simulink model "test_buoy_detector"  (Simulink 7.6)
settings: Solver=FixedStepDiscrete  StartTime=0.0  StopTime=0  RelTol=1e-3
undefined symbols (not defined in the file or in its folder): gray, jet, Rec, Scale_Forward_B, Scale_Forward_G, Scale_Forward_H, Scale_Forward_R, Scale_Forward_S, Scale_Forward_V, SDTV
libraries: vipsnks x10, vipconversions x3, viptextngfix x2, vipsrcs x1, dspmtrx3 x1
settings Model: Creator=Thing 1  LastModifiedBy=auvt
settings RTWCC: TargetLang=C++

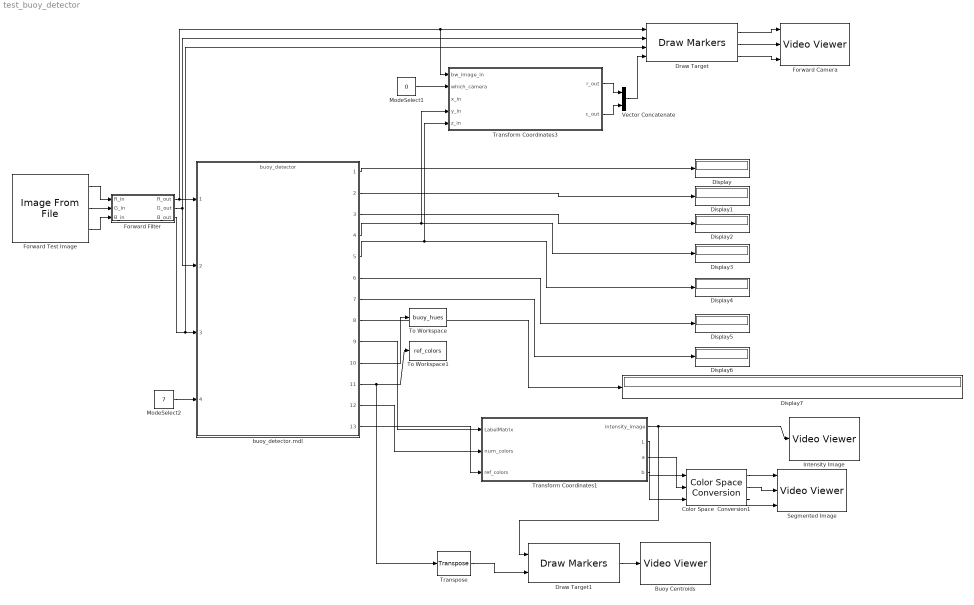
== system test_buoy_detector ==
  Buoy Centroids : vipsnks/Video Viewer  DialogControllerArgs=DataTag1  inputType=Obsolete7b  imagePorts=One multidimensional signal  useColorMap=off  colormapValue=jet(256)  specRange=off  minInputVal=0  maxInputVal=255  FigPos=[667 795 353 256]  AxisZoom=on  trueSizedOnce=off  OpenAtMdlStart=on
  Color Space  Conversion1 : vipconversions/Color Space  Conversion  conversion=Obsolete  conversionActive=L*a*b* to sR'G'B'  wp_str=D50  rec=Rec. 601 (SDTV)  sys=1125/60/2:1  imagePorts=Separate color signals
  Display{,1..7} (8 alike) : Display
  Draw Target : viptextngfix/Draw Markers  DialogController=vipDDGCreate  DialogControllerArgs=DataTag2  shape=X-mark  size=7  fill=off  fillClrSource=Specify via dialog  display=User-specified value  intensity=200  color=[0 0 0]  opacity=0.6  viewport=Entire image  antialiasing=off  inType=Obsolete  imagePorts=Separate color signals  prodOutputMode=Binary point scaling  prodOutputWordLength=32  prodOutputFracLength=14  memoryMode=Specify word length  memoryWordLength=16  memoryFracLength=15  roundingMode=Floor  overflowMode=off
  Draw Target1 : viptextngfix/Draw Markers  DialogController=vipDDGCreate  DialogControllerArgs=DataTag3  shape=X-mark  size=7  fill=off  fillClrSource=Specify via dialog  display=User-specified value  intensity=200  color=0  opacity=0.6  viewport=Entire image  antialiasing=off  inType=Obsolete  imagePorts=One multidimensional signal  prodOutputMode=Binary point scaling  prodOutputWordLength=32  prodOutputFracLength=14  memoryMode=Specify word length  memoryWordLength=16  memoryFracLength=15  roundingMode=Floor  overflowMode=off
  Forward Camera : vipsnks/Video Viewer  DialogControllerArgs=DataTag5  inputType=Obsolete7b  imagePorts=Separate color signals  useColorMap=off  colormapValue=jet(256)  specRange=off  minInputVal=0  maxInputVal=255  FigPos=[1090 387 268 224]  AxisZoom=on  trueSizedOnce=off  OpenAtMdlStart=on
  Forward Filter : Subsystem
  Forward Test Image : vipsrcs/Image From File  Tag=vipblks_nd  DialogController=vipDDGCreate  DialogControllerArgs=DataTag18  SystemSampleTime=-1  FileName=/home/auvt/auvc/src/vision/Test_Images/buoy6.PNG  imagePorts=Separate color signals  Ts=-1  ImageDataType=double  Signed=on  WordLength=16  sdImageDataType=uint(8)  FractionLengthMode=User-defined  FractionLength=15  OutPortLabels=R|G|B
  Intensity Image : vipsnks/Video Viewer  DialogControllerArgs=DataTag20  inputType=Obsolete7b  imagePorts=One multidimensional signal  useColorMap=off  colormapValue=jet(256)  specRange=off  minInputVal=0  maxInputVal=255  FigPos=[762 409 330 246]  AxisZoom=on  trueSizedOnce=off  OpenAtMdlStart=on
  ModeSelect1 : Constant  Value=0  SampleTime=-1
  ModeSelect2 : Constant  Value=7  SampleTime=-1
  Segmented Image : vipsnks/Video Viewer  DialogControllerArgs=DataTag22  inputType=Obsolete7b  imagePorts=Separate color signals  useColorMap=off  colormapValue=jet(256)  specRange=off  minInputVal=0  maxInputVal=255  FigPos=[957 848 410 300]  AxisZoom=on  trueSizedOnce=off  OpenAtMdlStart=on
  To Workspace : ToWorkspace  VariableName=buoy_hues  SampleTime=-1  SaveFormat=Array
  To Workspace1 : ToWorkspace  VariableName=ref_colors  SampleTime=-1  SaveFormat=Array
  Transform Coordinates1 : Stateflow chart  TreatAsAtomicUnit=on  SystemSampleTime=[1/30 0]
  Transform Coordinates3 : Stateflow chart  TreatAsAtomicUnit=on  SystemSampleTime=[1/30 0]
  Transpose : dspmtrx3/Transpose  SystemSampleTime=-1  Hermitian=off  overflowFlag=off
  Vector Concatenate : Concatenate  Mode=Multidimensional array
  buoy_detector.mdl : ModelReference  ModelNameDialog=buoy_detector  SimulationMode=Accelerator  ModelReferenceVersion=1.787  CopyOfModelName=buoy_detector
  wires:
  Forward Test Image/1 -> Forward Filter/1(R_in)
  Forward Test Image/3 -> Forward Filter/3(B_in)
  Vector Concatenate/1 -> Draw Target/4
  Draw Target/2 -> Forward Camera/2
  Draw Target/1 -> Forward Camera/1
  Draw Target/3 -> Forward Camera/3
  Forward Test Image/2 -> Forward Filter/2(G_in)
  ModeSelect1/1 -> Transform Coordinates3/2(which_camera)
  Transform Coordinates3/1(r_out) -> Vector Concatenate/1
  Transform Coordinates3/2(c_out) -> Vector Concatenate/2
  buoy_detector.mdl/1 -> Display/1
  buoy_detector.mdl/2 -> Display1/1
  buoy_detector.mdl/3 -> Display2/1
  buoy_detector.mdl/4 -> Display3/1, Transform Coordinates3/4(y_in)
  buoy_detector.mdl/5 -> Display4/1, Transform Coordinates3/5(z_in)
  buoy_detector.mdl/6 -> Display5/1
  buoy_detector.mdl/7 -> Display6/1
  buoy_detector.mdl/8 -> Display7/1
  ModeSelect2/1 -> buoy_detector.mdl/4
  Transform Coordinates1/1(intensity_image) -> Intensity Image/1, Draw Target1/1
  buoy_detector.mdl/10 -> To Workspace/1
  buoy_detector.mdl/11 -> To Workspace1/1, Transpose/1
  Draw Target1/1 -> Buoy Centroids/1
  Transpose/1 -> Draw Target1/2
  buoy_detector.mdl/12 -> Transform Coordinates1/2(num_colors)
  Transform Coordinates1/2(L) -> Color Space  Conversion1/1
  Transform Coordinates1/3(a) -> Color Space  Conversion1/2
  Transform Coordinates1/4(b) -> Color Space  Conversion1/3
  Color Space  Conversion1/1 -> Segmented Image/1
  Color Space  Conversion1/2 -> Segmented Image/2
  Color Space  Conversion1/3 -> Segmented Image/3
  Forward Filter/1(R_out) -> buoy_detector.mdl/1, Draw Target/1, Transform Coordinates3/1(bw_image_in)
  Forward Filter/2(G_out) -> buoy_detector.mdl/2, Draw Target/2
  Forward Filter/3(B_out) -> buoy_detector.mdl/3, Draw Target/3
  buoy_detector.mdl/9 -> Transform Coordinates1/1(LabelMatrix)
  buoy_detector.mdl/13 -> Transform Coordinates1/3(ref_colors)

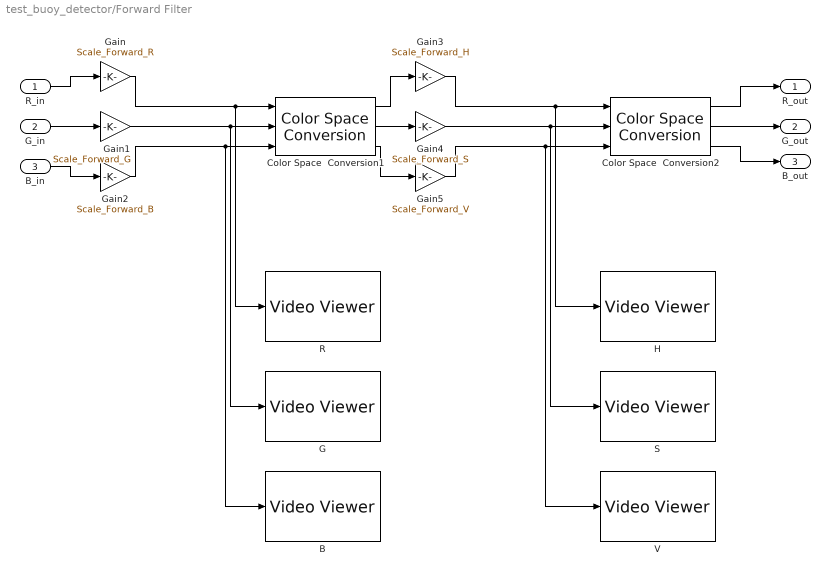
== system test_buoy_detector/Forward Filter ==
  R_in : Inport  PortDimensions=Forward_Camera_Dimensions
  G_in : Inport  Port=2  PortDimensions=Forward_Camera_Dimensions
  B_in : Inport  Port=3  PortDimensions=Forward_Camera_Dimensions
  B : vipsnks/Video Viewer  DialogControllerArgs=DataTag7  inputType=Obsolete7b  imagePorts=One multidimensional signal  useColorMap=off  colormapValue=gray(256)  specRange=off  minInputVal=0  maxInputVal=255  FigPos=[-59 861 410 300]  AxisZoom=on  trueSizedOnce=off  OpenAtMdlStart=on
  Color Space  Conversion1 : vipconversions/Color Space  Conversion  conversion=Obsolete  conversionActive=R'G'B' to HSV  wp_str=D50  rec=Rec. 601 (SDTV)  sys=1125/60/2:1  imagePorts=Separate color signals
  Color Space  Conversion2 : vipconversions/Color Space  Conversion  conversion=Obsolete  conversionActive=HSV to R'G'B'  wp_str=D50  rec=Rec. 601 (SDTV)  sys=1125/60/2:1  imagePorts=Separate color signals
  G : vipsnks/Video Viewer  DialogControllerArgs=DataTag9  inputType=Obsolete7b  imagePorts=One multidimensional signal  useColorMap=off  colormapValue=gray(256)  specRange=off  minInputVal=0  maxInputVal=255  FigPos=[-76 583 410 300]  AxisZoom=on  trueSizedOnce=off  OpenAtMdlStart=on
  Gain : Gain  Gain=Scale_Forward_R
  Gain1 : Gain  Gain=Scale_Forward_G
  Gain2 : Gain  Gain=Scale_Forward_B
  Gain3 : Gain  Gain=Scale_Forward_H
  Gain4 : Gain  Gain=Scale_Forward_S
  Gain5 : Gain  Gain=Scale_Forward_V
  H : vipsnks/Video Viewer  DialogControllerArgs=DataTag11  inputType=Obsolete7b  imagePorts=One multidimensional signal  useColorMap=off  colormapValue=gray(256)  specRange=off  minInputVal=0  maxInputVal=255  FigPos=[262 436 410 300]  AxisZoom=on  trueSizedOnce=off  OpenAtMdlStart=on
  R : vipsnks/Video Viewer  DialogControllerArgs=DataTag13  inputType=Obsolete7b  imagePorts=One multidimensional signal  useColorMap=off  colormapValue=gray(256)  specRange=off  minInputVal=0  maxInputVal=255  FigPos=[-86 436 410 300]  AxisZoom=on  trueSizedOnce=off  OpenAtMdlStart=on
  S : vipsnks/Video Viewer  DialogControllerArgs=DataTag15  inputType=Obsolete7b  imagePorts=One multidimensional signal  useColorMap=off  colormapValue=gray(256)  specRange=off  minInputVal=0  maxInputVal=255  FigPos=[253 614 410 300]  AxisZoom=on  trueSizedOnce=off  OpenAtMdlStart=on
  V : vipsnks/Video Viewer  DialogControllerArgs=DataTag17  inputType=Obsolete7b  imagePorts=One multidimensional signal  useColorMap=off  colormapValue=gray(256)  specRange=off  minInputVal=0  maxInputVal=255  FigPos=[249 894 410 300]  AxisZoom=on  trueSizedOnce=off  OpenAtMdlStart=on
  R_out : Outport  OutDataTypeStr=double
  G_out : Outport  Port=2  OutDataTypeStr=double
  B_out : Outport  Port=3  OutDataTypeStr=double
  wires:
  R_in/1 -> Gain/1
  G_in/1 -> Gain1/1
  B_in/1 -> Gain2/1
  Gain/1 -> Color Space  Conversion1/1, R/1
  Gain1/1 -> Color Space  Conversion1/2, G/1
  Gain2/1 -> Color Space  Conversion1/3, B/1
  Color Space  Conversion1/1 -> Gain3/1
  Color Space  Conversion1/2 -> Gain4/1
  Color Space  Conversion1/3 -> Gain5/1
  Gain3/1 -> Color Space  Conversion2/1, H/1
  Gain4/1 -> Color Space  Conversion2/2, S/1
  Gain5/1 -> Color Space  Conversion2/3, V/1
  Color Space  Conversion2/1 -> R_out/1
  Color Space  Conversion2/2 -> G_out/1
  Color Space  Conversion2/3 -> B_out/1

== matlab function Transform Coordinates3 ==
  data: bw_image_in input double; which_camera input double; x_in input double; y_in input double; r_out output double; c_out output double; z_in input double
function [r_out, c_out] = transform_G2L(bw_image_in, which_camera, x_in, y_in, z_in)
% This function, "transform Global to Local coordinates," transforms
%   global coordinates that are sent to the controller into local
%   coordinates that can be displayed over images.
%
% 5-29-11
%
% Input
%   x_in, y_in, z_in = vectors of points in global (vehicle-centered)
%     coordinate system
%   bw_image_in = a 2-D array of pixel values (used only to extract image
%     size)
%   which_camera = selects which camera for relative coordinates
%                = 0 -> Forward camera
%                = 1 -> Down camera
%
% Output
%   r_out, c_out = row, column pairs in local coordinate system

[rows, cols] = size(bw_image_in);
if( which_camera == 0 )
    r_out = z_in + floor(rows/2);
    c_out = y_in + floor(cols/2);
else
    r_out = floor(rows/2) - x_in;
    c_out = y_in + floor(cols/2);
end

return

== matlab function Transform Coordinates1 ==
  data: LabelMatrix input double; intensity_image output double; num_colors input double; ref_colors input double; L output double; a output double; b output double
function [intensity_image, L, a, b] = displaySegmentedImage(LabelMatrix, num_colors, ref_colors)


intensity_image = LabelMatrix./max(max(max(abs(LabelMatrix))));


[rows, cols] = size(LabelMatrix);

L = zeros(rows, cols);
a = zeros(rows, cols);
b = zeros(rows, cols);

for r = 1:rows
    for c = 1:cols
        L(r,c) = ref_colors(LabelMatrix(r,c), 1);
        a(r,c) = ref_colors(LabelMatrix(r,c), 2);
        b(r,c) = ref_colors(LabelMatrix(r,c), 3);
    end
end

return
